simulink model "PIC32MK_MCPWM_MCLV2_PIM_SingleShunt_R2015b_InternalOpAmp"  (R2015b)
settings: Solver=FixedStepDiscrete  StartTime=0.0  StopTime=1  FixedStep=5e-5  RelTol=1e-3
undefined symbols (not defined in the file): A0, A11, A4, AN24, AN25, AN6, AN9, B6, B7, B9, C0, C8, DiscIntNeverNeededParam, G15, MaxPer, ms, Pin, PWM1max, Resol, us, XData
libraries: MCHP_Blockset x14, simulink x9
(part 3 of 3)

== system PIC32MK_MCPWM_MCLV2_PIM_SingleShunt_R2015b_InternalOpAmp/Sliding Mode Observer1/Atan x2/abs ==
  In3 : Inport
  Compare To Zero : simulink/Logic and Bit Operations/Compare To Zero  relop=>=  OutDataTypeStr=boolean
  Gain : Gain  Gain=-1  OutDataTypeStr=Inherit: Same as input
  Switch2 : Switch  Criteria=u2 ~= 0
  abs : Outport
  sign : Outport  Port=2
  wires:
  Compare To Zero/1 -> Switch2/2, sign/1
  In3/1 -> Compare To Zero/1, Switch2/1, Gain/1
  Gain/1 -> Switch2/3
  Switch2/1 -> abs/1

== system PIC32MK_MCPWM_MCLV2_PIM_SingleShunt_R2015b_InternalOpAmp/Sliding Mode Observer1/Atan x2/abs1 ==
  In3 : Inport
  Compare To Zero : simulink/Logic and Bit Operations/Compare To Zero  relop=>=  OutDataTypeStr=boolean
  Gain : Gain  Gain=-1  OutDataTypeStr=Inherit: Same as input
  Switch2 : Switch  Criteria=u2 ~= 0
  abs : Outport
  sign : Outport  Port=2
  wires:
  Switch2/1 -> abs/1
  Gain/1 -> Switch2/3
  In3/1 -> Gain/1, Switch2/1, Compare To Zero/1
  Compare To Zero/1 -> sign/1, Switch2/2

== system PIC32MK_MCPWM_MCLV2_PIM_SingleShunt_R2015b_InternalOpAmp/Sliding Mode Observer1/SMO FxPt/Clark1 ==
  note: k = 2/3 : invariant Magnitude
  note: Input is a vector of 3 elements, 3rd element is not beeing used
  ab(c) : Inport
  Clarke1 : Product  Multiplication=Matrix(*)  OutMin=[-4.4]  OutMax=[4.4]  OutDataTypeStr=fixdt(1,16)  SaturateOnIntegerOverflow=on  RndMeth=Zero
  Constant Magnitude : Constant  Value=[1 0 ; 1/sqrt(3) 2/sqrt(3) ];  OutDataTypeStr=fixdt(1,16)
  Data Type Conversion : DataTypeConversion  RndMeth=Zero
  Demux1 : Demux  Outputs=2
  Gain1 : Gain  Gain=1/sqrt(3)  OutMin=[-4.4]  OutMax=[4.4]  OutDataTypeStr=double  RndMeth=Zero
  Gain2 : Gain  Gain=2/sqrt(3)  OutMin=[-4.4]  OutMax=[4.4]  OutDataTypeStr=double  RndMeth=Zero
  Mux1 : Mux  Inputs=2
  Sum2 : Sum  RndMeth=Zero  OutDataTypeStr=Inherit: Same as first input
  alpha beta : Outport
  wires:
  Data Type Conversion/1 -> Mux1/1
  Mux1/1 -> alpha beta/1
  Sum2/1 -> Mux1/2
  Gain2/1 -> Sum2/2
  Gain1/1 -> Sum2/1
  Demux1/2 -> Gain2/1
  Demux1/1 -> Data Type Conversion/1, Gain1/1
  Constant Magnitude/1 -> Clarke1/1
  ab(c)/1 -> Clarke1/2, Demux1/1
